simulink model "deneme4"  (R2023b)
settings: Solver=VariableStepAuto  StartTime=0.0  StopTime=10.0  RelTol=1e-3
settings Model: Creator=SafakPC  LastModifiedBy=SafakPC

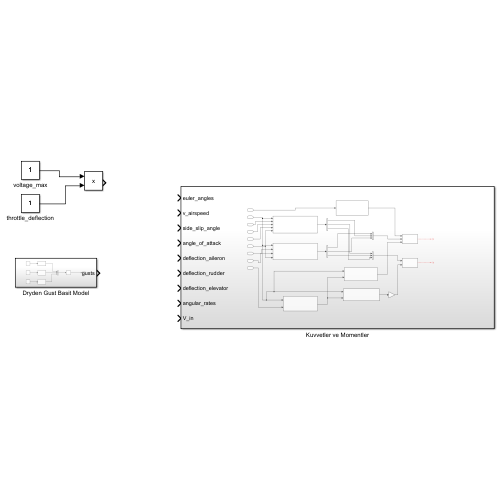
[thumbnail: Simulink's stored preview of the top-level diagram]
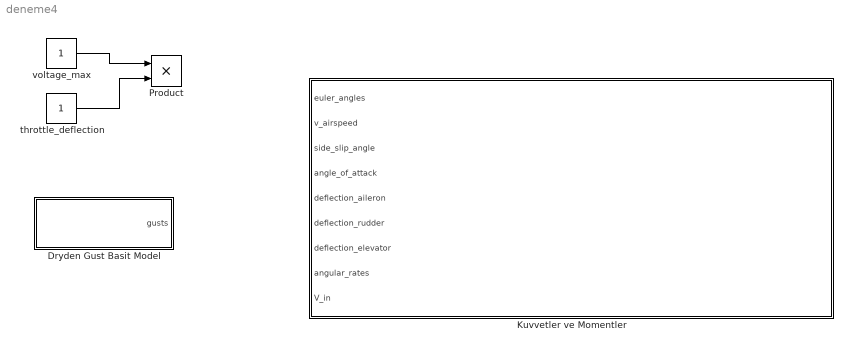
== system deneme4 ==
  Dryden Gust Basit Model : Subsystem
  Kuvvetler ve Momentler : Subsystem
  Product : Product
  throttle_deflection : Constant
  voltage_max : Constant
  wires:
  voltage_max/1 -> Product/1
  throttle_deflection/1 -> Product/2

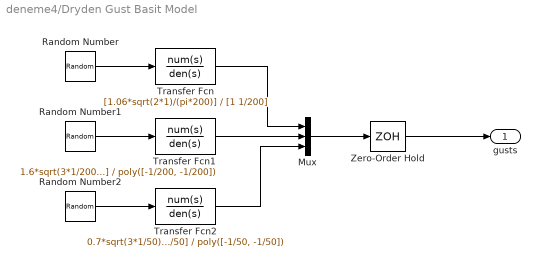
== system deneme4/Dryden Gust Basit Model ==
  Mux : Mux  Inputs=3
  Random Number : RandomNumber  SampleTime=0
  Random Number1 : RandomNumber  SampleTime=0
  Random Number2 : RandomNumber  SampleTime=0
  Transfer Fcn : TransferFcn  Numerator=[1.06*sqrt(2*1)/(pi*200)]  Denominator=[1 1/200]
  Transfer Fcn1 : TransferFcn  Numerator=1.6*sqrt(3*1/200)*[0, 1, 1/sqrt(3)/200]  Denominator=poly([-1/200, -1/200])
  Transfer Fcn2 : TransferFcn  Numerator=0.7*sqrt(3*1/50)*[0, 1, 1/sqrt(3)/50]  Denominator=poly([-1/50, -1/50])
  Zero-Order Hold : ZeroOrderHold  SampleTime=-1
  gusts : Outport
  wires:
  Random Number/1 -> Transfer Fcn/1
  Random Number1/1 -> Transfer Fcn1/1
  Random Number2/1 -> Transfer Fcn2/1
  Transfer Fcn/1 -> Mux/1
  Transfer Fcn1/1 -> Mux/2
  Transfer Fcn2/1 -> Mux/3
  Mux/1 -> Zero-Order Hold/1
  Zero-Order Hold/1 -> gusts/1

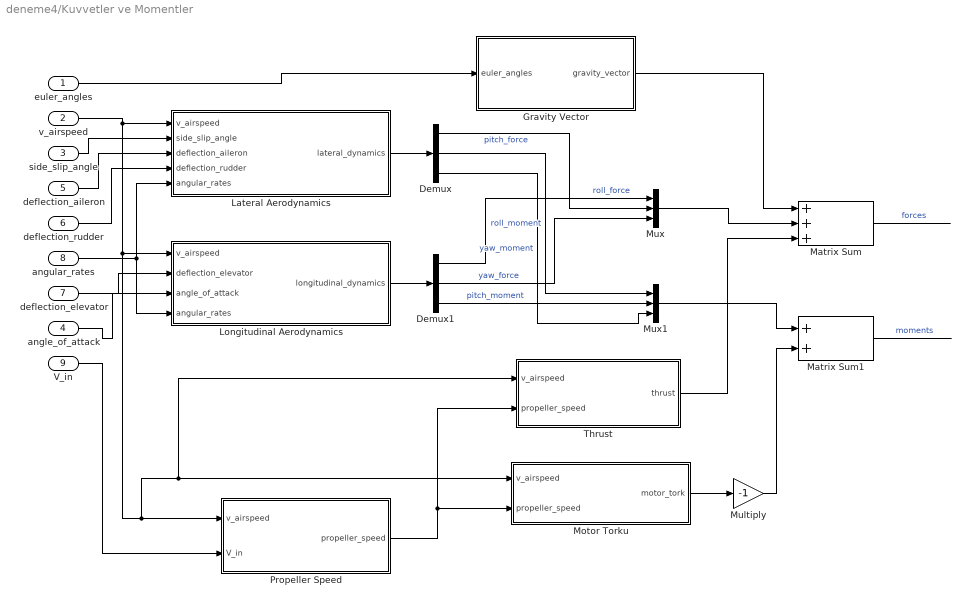
== system deneme4/Kuvvetler ve Momentler ==
  euler_angles : Inport
  v_airspeed : Inport  Port=2
  side_slip_angle : Inport  Port=3
  angle_of_attack : Inport  Port=4
  deflection_aileron : Inport  Port=5
  deflection_rudder : Inport  Port=6
  deflection_elevator : Inport  Port=7
  angular_rates : Inport  Port=8
  V_in : Inport  Port=9
  Demux : Demux  Outputs=3
  Demux1 : Demux  Outputs=3
  Gravity Vector : MATLAB Function  TreatAsAtomicUnit=on
  Lateral Aerodynamics : MATLAB Function  TreatAsAtomicUnit=on
  Longitudinal Aerodynamics : MATLAB Function  TreatAsAtomicUnit=on
  Matrix Sum : Sum  Inputs=+++
  Matrix Sum1 : Sum
  Motor Torku : MATLAB Function  TreatAsAtomicUnit=on
  Multiply : Gain  Gain=-1
  Mux : Mux  Inputs=3
  Mux1 : Mux  Inputs=3
  Propeller Speed : MATLAB Function  TreatAsAtomicUnit=on
  Thrust : MATLAB Function  TreatAsAtomicUnit=on
  wires:
  deflection_rudder/1 -> Lateral Aerodynamics/4(deflection_rudder)
  deflection_aileron/1 -> Lateral Aerodynamics/3(deflection_aileron)
  angular_rates/1 -> Lateral Aerodynamics/5(angular_rates), Longitudinal Aerodynamics/4(angular_rates)
  euler_angles/1 -> Gravity Vector/1(euler_angles)
  deflection_elevator/1 -> Longitudinal Aerodynamics/2(deflection_elevator)
  angle_of_attack/1 -> Longitudinal Aerodynamics/3(angle_of_attack)
  Lateral Aerodynamics/1(lateral_dynamics) -> Demux/1
  Demux/1 -> Mux/2  "pitch_force"
  Demux/2 -> Mux1/1  "roll_moment"
  Longitudinal Aerodynamics/1(longitudinal_dynamics) -> Demux1/1
  Demux/3 -> Mux1/3  "yaw_moment"
  Demux1/1 -> Mux/1  "roll_force"
  Demux1/2 -> Mux/3  "yaw_force"
  Demux1/3 -> Mux1/2  "pitch_moment"
  Mux/1 -> Matrix Sum/2
  v_airspeed/1 -> Thrust/1(v_airspeed), Motor Torku/1(v_airspeed), Propeller Speed/1(v_airspeed), Longitudinal Aerodynamics/1(v_airspeed), Lateral Aerodynamics/1(v_airspeed)
  V_in/1 -> Propeller Speed/2(V_in)
  Motor Torku/1(motor_tork) -> Multiply/1
  Thrust/1(thrust) -> Matrix Sum/3
  Propeller Speed/1(propeller_speed) -> Thrust/2(propeller_speed), Motor Torku/2(propeller_speed)
  Gravity Vector/1(gravity_vector) -> Matrix Sum/1
  Matrix Sum/1 -> ?  "forces"
  Mux1/1 -> Matrix Sum1/1
  Multiply/1 -> Matrix Sum1/2
  Matrix Sum1/1 -> ?  "moments"
  side_slip_angle/1 -> Lateral Aerodynamics/2(side_slip_angle)

== matlab function deneme4/Kuvvetler ve Momentler/Propeller Speed ==
  data: propeller_speed output; v_airspeed input; V_in input
function propeller_speed = fcn(v_airspeed, V_in)

%model parametreleri
air_density = 0;
prop_diameter = 0;
internal_resistance = 0;
no_load_current = 0;
KQ = 0; KV = 0; CQ0 = 0; CQ1 = 0; CQ2 = 0;






a = (((air_density * (prop_diameter^5)) / ((2 * pi)*(2 * pi))) * CQ0);
b = ((((air_density * (prop_diameter^4)) / (2*pi)) * (CQ1 * v_airspeed)) + ((KQ*KV) / internal_resistance));
c = (air_density * (prop_diameter^3) * CQ2 * v_airspeed * v_airspeed) - ((KQ/R)*V_in) + (KQ * no_load_current);

omega_P = (-b + sqrt(((b*b)-4*a*c))) / 2*a;

propeller_speed = omega_P;

end

== matlab function deneme4/Kuvvetler ve Momentler/Gravity Vector ==
  data: gravity_vector output; euler_angles input
function gravity_vector = fcn(euler_angles)

    %model parametresi = aerosonde
    mass = 0;

    %yerçekimi vektörünün hesaplanması
    phi = euler_angles(1);
    theta = euler_angles(2);
    psi = euler_angles(3);
    gravity_constant = 9.81;

    a11 = (-mass*gravity_constant*sin(theta));
    a21 = (mass*gravity_constant*cos(theta)*sin(phi));
    a31 = (mass*gravity_constant*cos(theta)*cos(phi));

    gravity_vector = [a11;a21;a31];
    
end

== matlab function deneme4/Kuvvetler ve Momentler/Thrust ==
  data: thrust output; v_airspeed input; propeller_speed input
function thrust = fcn(v_airspeed,propeller_speed)
%model parametreleri - aerosonde
air_density = 0;
prop_diameter = 0;
CT0 = 0; CT1 = 0; CT2 = 0;
Tp_p1 = ((air_density * (prop_diameter^4) * CT0) / (4 * pi * pi)) * propeller_speed * propeller_speed;
Tp_p2 = ((air_density * (prop_diameter^3) * CT1 * v_airspeed) / (2*pi)) * propeller_speed;
Tp_p3 = (air_density * (prop_diameter^2) * CT2 * v_airspeed * v_airspeed);

Tp = Tp_p1 + Tp_p2 + Tp_p3;

thrust = [Tp;0;0];

end

== matlab function deneme4/Kuvvetler ve Momentler/Motor Torku ==
  data: motor_tork output; v_airspeed input; propeller_speed input
function motor_tork = fcn(v_airspeed,propeller_speed)
%model parametreleri - aerosonde
air_density = 0;
prop_diameter = 0;
CQ0 = 0; CQ1 = 0; CQ2 = 0;

Qp_p1 = ((air_density * (prop_diameter^5) * CQ0) / (4 * pi * pi)) * propeller_speed * propeller_speed;
Qp_p2 = ((air_density * (prop_diameter^4) * CQ1 * v_airspeed) / (2*pi)) * propeller_speed;
Qp_p3 = (air_density * (prop_diameter^3) * CQ2 * v_airspeed * v_airspeed);

Qp = Qp_p1 + Qp_p2 + Qp_p3;

motor_tork = [Qp;0;0];

end

== matlab function deneme4/Kuvvetler ve Momentler/Lateral Aerodynamics ==
  data: v_airspeed input; side_slip_angle input; lateral_dynamics output; deflection_aileron input; deflection_rudder input; angular_rates input
function lateral_dynamics = fcn(v_airspeed, side_slip_angle, deflection_aileron, deflection_rudder, angular_rates)
%model parametreleri - aerosonde
p = angular_rates(1);
r = angular_rates(3);
air_density = 0; 
wing_surface_area = 0;
wing_span = 4; 

CY0 = 0; CYB = 0; CYP = 0; CYR = 0; CYDA = 0; CYDR = 0;
Cl0 = 0; ClB = 0; ClP = 0; ClR = 0; ClDA = 0; ClDR = 0;
Cn0 = 0; CnB = 0; CnP = 0; CnR = 0; CnDA = 0; CnDR = 0;


var1 = (0.5 * air_density * (v_airspeed^2) * wing_surface_area);
lateral_force = var1 * (CY0 + (CYB*side_slip_angle) + (CYP * ((wing_span/2*v_airspeed)*p))+(CYR * ((wing_span/2*v_airspeed) * r)) + (CYDA * deflection_aileron) + (CYDR * deflection_rudder));
roll_moment = (var1 * wing_span)*(Cl0 + (ClB*side_slip_angle) + (ClP * ((wing_span/2*v_airspeed)*p))+(ClR * ((wing_span/2*v_airspeed) * r)) + (ClDA * deflection_aileron) + (ClDR * deflection_rudder));
yaw_moment = (var1 * wing_span)*(Cn0 + (CnB*side_slip_angle) + (CnP * ((wing_span/2*v_airspeed)*p))+(CnR * ((wing_span/2*v_airspeed) * r)) + (CnDA * deflection_aileron) + (CnDR * deflection_rudder));
lateral_dynamics = [lateral_force;roll_moment;yaw_moment];

end

== matlab function deneme4/Kuvvetler ve Momentler/Longitudinal Aerodynamics ==
  data: v_airspeed input; deflection_elevator input; angle_of_attack input; longitudinal_dynamics output; angular_rates input
function longitudinal_dynamics = fcn(v_airspeed, deflection_elevator, angle_of_attack,   angular_rates)
p = angular_rates(1);
q = angular_rates(2);
r = angular_rates(3);

%model parametereleri - aerosonde
transition_rate = 50; aoa0 = 0.47;
eos = 0.9; CL0 = 0.23; CDp = 0.043; CDq = 0; CLq = 7.95;
CLDe = 0.13; CDDe = 0.0135; 
wing_span = 0; wing_surface_area = 0;
air_density = 0; mean_chord = 0;
CM0 = 0; CMa = 0; CMq = 0 ; CMDe = 0;

%lift katsayısının hesaplanması
aspect_ratio = ((wing_span*wing_span) / wing_surface_area);
CL_alpha = (pi*aspect_ratio) / (1+root(1+((aspect_ratio/2)*(aspect_ratio/2))));
CL_flatplate = 2 * sign(angle_of_attack) * sin(angle_of_attack) * sin(angle_of_attack) * cos(angle_of_attack);
var1 = -(transition_rate * (angle_of_attack - aoa0));
var2 = (transition_rate * (angle_of_attack + aoa0));
sigmoid_alpha =  ( 1 + exp(var1) + exp(var2) ) / ( (1 + exp(var1)) * (1 + exp(var2)) );
CL = ((1-sigmoid_alpha)*(CL0 + (angle_of_attack * CL_alpha))) + (sigmoid_alpha*CL_flatplate);

%drag katsayısının hesaplanması
CD = CDp + (((CL_alpha * angle_of_attack)^2) / (pi * eos * aspect_ratio));

%diğer parametrelerin hesaplanması
CX = (-CD * cos(angle_of_attack)) + (CL * sin(angle_of_attack));
CXq = (-CDq * cos(angle_of_attack)) + (CLq * sin(angle_of_attack));
CXDe = (-CDDe * cos(angle_of_attack)) + (CLDe * sin(angle_of_attack));
CZ = (-CD * sin(angle_of_attack)) - (CL * cos(angle_of_attack));
CZq = (-CDq * sin(angle_of_attack)) - (CLq * cos(angle_of_attack));
CZDe = (-CDDe * sin(angle_of_attack)) - (CLDe * cos(angle_of_attack));

%kuvvet ve momentlerin hesaplanması
var1 = (0.5 * air_density * (v_airspeed^2) * wing_surface_area);
roll_force = var1 * (CX + (CXq * ((mean_chord/2*v_airspeed)*q))+ (CXDe * deflection_elevator));
yaw_force = var1 * (CZ + (CZq * ((mean_chord/2*v_airspeed)*q))+ (CZDe * deflection_elevator));
pitch_moment = (var1 *  mean_chord)*(CM0 + (CMa * angle_of_attack) + (CMq * (mean_chord/2*v_airspeed)*q)) + (CMDe * deflection_elevator);
longitudinal_dynamics = [roll_force;yaw_force;pitch_moment];

end
